simulink model "switching_controller_parallel_before_retraining"  (R2020a)
settings: Solver=FixedStepAuto  StartTime=0.0  StopTime=simulation.time_window  FixedStep=simulation.time_step  MaxStep=.2  RelTol=1e-3
model workspace (MAT data in the model file):
  PID_TRESH = 0.3
undefined symbols (not defined in the file): DiscIntNeverNeededParam
libraries: neural x36, simulink x1
(part 2 of 2)

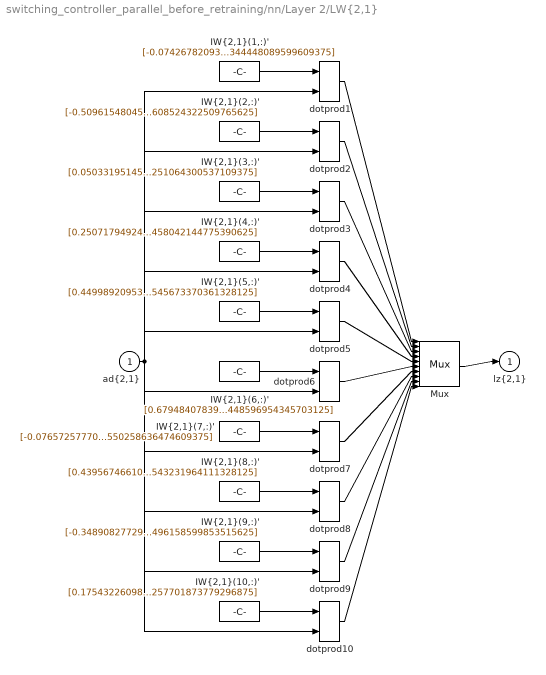
== system switching_controller_parallel_before_retraining/nn/Layer 2/LW{2,1} ==
  "ad{2,1}" : Inport  PortDimensions=20
      mask Display: e = 0.06;c1 = [120 230 180]/255;c2 = ([120 230 180]+0)/(256+128);c3 = ([120 230 180]+128)/(256+128);patch([0 1 1 0],[0 0 1 1],c1);patch([0 1 1 1-e 1-e 0+e],[0 0 1 1-e 0+e 0+e],c2);patch([0 0 1 1-e 0+e 0+e],[0 1 1 1-e 1-e 0+e],c3);plot([0 1 1 0 0],[0 0 1 1 0]);
  "IW{2,1}(1,:)'" : Constant  Value=[-0.0742678209385321530522361399562214501202106475830078125;-0.25241332220814294284849665928049944341182708740234375;0.1582652995009124208269923883563023991882801055908203125;0.0409941814809637872230041466536931693553924560546875;0.1777509687795489623507450005490682087838649749755859375;-0.56378494502083043027340636399458162486553192138671875;-0.52966898056344147160956481457105837762355804443359375;-0.5491849542615752088892122628749348223209381103515625;-0.366642992817404422822846754570491611957550048828125;-0.30113881397149777630062317257397808134555816650390625;0.36352811076936453194008436184958554804325103759765625;-0.5626667254561283915137437361408956348896026611328125;0.27233462192782542654612143451231531798839569091796875;-0.137529463271337970553531704354099929332733154296875;0.2251042526934673160265987235106877051293849945068359375;-0.267991412908181458885081838161568157374858856201171875;0.0487266727373815433654868911617086268961429595947265625;0.52897529061972725639151349241728894412517547607421875;0.08173542337008686542443314237971208058297634124755859375;-0.72183912669657279703727681408054195344448089599609375]
      mask Display: e = 0.06;c1 = [120 150 230]/255;c2 = ([120 150 230]+0)/383;c3 = ([120 150 230]+128)/383;patch([0 1 1 0],[0 0 1 1],c1);patch([0 1 1 1-e 1-e 0+e],[0 0 1 1-e 0+e 0+e],c2);patch([0 0 1 1-e 0+e 0+e],[0 1 1 1-e 1-e 0+e],c3);plot([0 1 1 0 0],[0 0 1 1 0]);disp('weights');
  "IW{2,1}(10,:)'" : Constant  Value=[0.1754322609814331357380723375172237865626811981201171875;0.33947484743859224209927560877986252307891845703125;0.322169525908290677040923810636741109192371368408203125;-0.5029839312713904053708802166511304676532745361328125;0.376908084486362648934942853884422220289707183837890625;-0.19411578487550318339316390847670845687389373779296875;-0.472436961613329098330638089464628137648105621337890625;-0.4250614998526458521155291236937046051025390625;-0.321656192995510459287089588542585261166095733642578125;0.409800051137812537671578638764913193881511688232421875;0.1634407939921007635319938344764523208141326904296875;-0.1060868965133207331152931374163017608225345611572265625;-0.417317840820639773813383044398506172001361846923828125;0.53238420036386358002999941163579933345317840576171875;-0.271228839256366149879085014617885462939739227294921875;-0.390405815950181367401938814509776420891284942626953125;-0.35866328688225135312706015611183829605579376220703125;0.394312295760493702889704081826494075357913970947265625;0.464923085316455597659768272933433763682842254638671875;0.181321777068363221285807185267913155257701873779296875]
      mask Display: e = 0.06;c1 = [120 150 230]/255;c2 = ([120 150 230]+0)/383;c3 = ([120 150 230]+128)/383;patch([0 1 1 0],[0 0 1 1],c1);patch([0 1 1 1-e 1-e 0+e],[0 0 1 1-e 0+e 0+e],c2);patch([0 0 1 1-e 0+e 0+e],[0 1 1 1-e 1-e 0+e],c3);plot([0 1 1 0 0],[0 0 1 1 0]);disp('weights');
  "IW{2,1}(2,:)'" : Constant  Value=[-0.50961548045789861749454985329066403210163116455078125;-0.253176760952781965130498065263964235782623291015625;-0.436374658893074085508345660855411551892757415771484375;-0.058776816615726999726287971270721754990518093109130859375;-0.1343536738257948837116373397293500602245330810546875;-0.53904710028970426183292374844313599169254302978515625;0.52574685179374025523202362819574773311614990234375;-0.14503214797993979612300563530880026519298553466796875;-0.41610507400117657805793669467675499618053436279296875;0.2258338290688970129149737431362154893577098846435546875;0.452630270340266649409244337221025489270687103271484375;-0.3838510809241111321199468875420279800891876220703125;-0.080043804629484960333485332739655859768390655517578125;0.086988039921783444352598735349602065980434417724609375;-0.30566584836628951649117880151607096195220947265625;0.078603298531889131961492012123926542699337005615234375;-0.2146956389255603447896447733000968582928180694580078125;-0.49159733673330541225965362173155881464481353759765625;-0.07920516278329912951416957866968004964292049407958984375;-0.2297869666393469734178012231495813466608524322509765625]
      mask Display: e = 0.06;c1 = [120 150 230]/255;c2 = ([120 150 230]+0)/383;c3 = ([120 150 230]+128)/383;patch([0 1 1 0],[0 0 1 1],c1);patch([0 1 1 1-e 1-e 0+e],[0 0 1 1-e 0+e 0+e],c2);patch([0 0 1 1-e 0+e 0+e],[0 1 1 1-e 1-e 0+e],c3);plot([0 1 1 0 0],[0 0 1 1 0]);disp('weights');
  "IW{2,1}(3,:)'" : Constant  Value=[0.050331951453894137327171875995190930552780628204345703125;-0.1980455271011341000786387667176313698291778564453125;0.5464228112888898092336376066668890416622161865234375;0.143258734343598204130643125608912669122219085693359375;0.6545378931000180866561777293100021779537200927734375;0.0029693683728794183218635538423768593929708003997802734375;0.331210089212467140296070056137978099286556243896484375;-0.05628620519114226061763162078932509757578372955322265625;0.51382712775967875895588576895534060895442962646484375;-0.21961621362080319119769455937785096466541290283203125;0.6861028831776201375447499231086112558841705322265625;0.193895474485615337822963510916451923549175262451171875;-0.25453832761822337005241934093646705150604248046875;0.45117937720722867123157584501313976943492889404296875;-0.28569063753284329454373846601811237633228302001953125;-0.50475380514631817963078219690942205488681793212890625;-0.378178164082300261039648603400564752519130706787109375;-0.03749349210638715235166529282651026733219623565673828125;0.0239248285341571442774721845125895924866199493408203125;-0.4295334690027734492190347737050615251064300537109375]
      mask Display: e = 0.06;c1 = [120 150 230]/255;c2 = ([120 150 230]+0)/383;c3 = ([120 150 230]+128)/383;patch([0 1 1 0],[0 0 1 1],c1);patch([0 1 1 1-e 1-e 0+e],[0 0 1 1-e 0+e 0+e],c2);patch([0 0 1 1-e 0+e 0+e],[0 1 1 1-e 1-e 0+e],c3);plot([0 1 1 0 0],[0 0 1 1 0]);disp('weights');
  "IW{2,1}(4,:)'" : Constant  Value=[0.25071794924415391481176129673258401453495025634765625;-0.25655473735131739676518236592528410255908966064453125;-0.125932536431736907811540504553704522550106048583984375;0.2358601050679441646362732853958732448518276214599609375;-0.50129483332140190032788495955173857510089874267578125;-0.07287292485839162725635986816996592096984386444091796875;-0.349288031403435395016998654682538472115993499755859375;0.10293619314487244265077237059813342057168483734130859375;-0.10469867031949632585341447565951966680586338043212890625;-0.398005841630075518633447018146398477256298065185546875;1.2743088847126571305778952591936103999614715576171875;0.426094930489777201643164517008699476718902587890625;0.3634133834892663283966385279200039803981781005859375;-0.0288941994596689059882077543761624838225543498992919921875;-0.30862723401891811736419413136900402605533599853515625;0.4189583770900477954768348354264162480831146240234375;-0.1382079784576591141576074051044997759163379669189453125;-0.288297871213736012219186477523180656135082244873046875;0.224223812097748720351120255145360715687274932861328125;0.06845932428237412603611034001005464233458042144775390625]
      mask Display: e = 0.06;c1 = [120 150 230]/255;c2 = ([120 150 230]+0)/383;c3 = ([120 150 230]+128)/383;patch([0 1 1 0],[0 0 1 1],c1);patch([0 1 1 1-e 1-e 0+e],[0 0 1 1-e 0+e 0+e],c2);patch([0 0 1 1-e 0+e 0+e],[0 1 1 1-e 1-e 0+e],c3);plot([0 1 1 0 0],[0 0 1 1 0]);disp('weights');
  "IW{2,1}(5,:)'" : Constant  Value=[0.449989209535755441127236053944216109812259674072265625;0.1668938640746752966048660482556442730128765106201171875;-0.1528747166922375944064782515852130018174648284912109375;-0.466413182483166377512162625862401910126209259033203125;0.319019707786719119990692661303910426795482635498046875;-0.269682605526375407389849669925752095878124237060546875;-0.286146420418946723085440453360206447541713714599609375;-0.1124570366042244862203602906447486020624637603759765625;-0.60761075348500115378413966027437709271907806396484375;-0.09832625527147524635562803041466395370662212371826171875;0.416238919016751030000023092725314199924468994140625;0.41417684214283412291734975951840169727802276611328125;0.1285238721039599629758498622322804294526576995849609375;0.04150845561035156061624462608961039222776889801025390625;-0.5181335247944744981651865600724704563617706298828125;0.024835012212249894802962302264859317801892757415771484375;-0.370454183035626993802935658095520921051502227783203125;0.260088553967631863628184873959980905055999755859375;0.437350919400649795765190219754003919661045074462890625;-0.46632501805306703079878616335918195545673370361328125]
      mask Display: e = 0.06;c1 = [120 150 230]/255;c2 = ([120 150 230]+0)/383;c3 = ([120 150 230]+128)/383;patch([0 1 1 0],[0 0 1 1],c1);patch([0 1 1 1-e 1-e 0+e],[0 0 1 1-e 0+e 0+e],c2);patch([0 0 1 1-e 0+e 0+e],[0 1 1 1-e 1-e 0+e],c3);plot([0 1 1 0 0],[0 0 1 1 0]);disp('weights');
  "IW{2,1}(6,:)'" : Constant  Value=[0.679484078395458102050952220452018082141876220703125;0.04141787402921648375553331788978539407253265380859375;-0.07852831144106568739271523327261093072593212127685546875;-0.06946291361144722731335576781930285505950450897216796875;0.5862015780018110522320284871966578066349029541015625;0.008164688663760931441881751879918738268315792083740234375;0.01267656278289677578008376457319172914139926433563232421875;0.35129857330214397936885006856755353510379791259765625;-0.281716957188827610281123270397074520587921142578125;-0.377956077447295590854281499559874646365642547607421875;0.399883631711499820671207316991058178246021270751953125;0.421701849253063698608201548267970792949199676513671875;0.38087921164733506973476551138446666300296783447265625;-0.1444822361794708687199317864724434912204742431640625;-0.3082207979968611955001733804238028824329376220703125;0.52705156187305790549402217948227189481258392333984375;0.211120738453866751971332860193797387182712554931640625;0.64083647291273748702877810501377098262310028076171875;-0.33683964993104031915294171994901262223720550537109375;0.258659389379542137277212532353587448596954345703125]
      mask Display: e = 0.06;c1 = [120 150 230]/255;c2 = ([120 150 230]+0)/383;c3 = ([120 150 230]+128)/383;patch([0 1 1 0],[0 0 1 1],c1);patch([0 1 1 1-e 1-e 0+e],[0 0 1 1-e 0+e 0+e],c2);patch([0 0 1 1-e 0+e 0+e],[0 1 1 1-e 1-e 0+e],c3);plot([0 1 1 0 0],[0 0 1 1 0]);disp('weights');
  "IW{2,1}(7,:)'" : Constant  Value=[-0.0765725777039530097756170334832859225571155548095703125;0.045295261798219167703738463615081855095922946929931640625;0.120469739157076538571544688238645903766155242919921875;0.3880656334730634426932738278992474079132080078125;-0.175604394629628013380084894379251636564731597900390625;0.1717388843781173235480963512600283138453960418701171875;0.381286326232597894136944205456529743969440460205078125;0.511569138199252648746551130898296833038330078125;0.11038162503234556777176322839295607991516590118408203125;0.6655250283685323342552919712034054100513458251953125;-0.3652469434145084736798025915049947798252105712890625;0.07177631492141227365078037792045506648719310760498046875;0.069664886066460873781380769287352450191974639892578125;-0.432032970640127411687814174001687206327915191650390625;-0.583466461683132653348593521513976156711578369140625;0.55591735512564655063982854699133895337581634521484375;-0.270067076847661013960788523036171682178974151611328125;0.382977519217001127760369172392529435455799102783203125;0.264177680981460272224836671739467419683933258056640625;-0.1612088776390406541505484483423060737550258636474609375]
      mask Display: e = 0.06;c1 = [120 150 230]/255;c2 = ([120 150 230]+0)/383;c3 = ([120 150 230]+128)/383;patch([0 1 1 0],[0 0 1 1],c1);patch([0 1 1 1-e 1-e 0+e],[0 0 1 1-e 0+e 0+e],c2);patch([0 0 1 1-e 0+e 0+e],[0 1 1 1-e 1-e 0+e],c3);plot([0 1 1 0 0],[0 0 1 1 0]);disp('weights');
  "IW{2,1}(8,:)'" : Constant  Value=[0.439567466102353698875759846487198956310749053955078125;-0.55137685168932482060455413375166244804859161376953125;-0.29550672253545806622554437126382254064083099365234375;-0.036798516056060610879274719309250940568745136260986328125;-0.2344144146160440644877098748111166059970855712890625;-0.0033479905308381983919385760373188531957566738128662109375;0.457258477431225662801494991072104312479496002197265625;0.1756065159579283940782801209934405051171779632568359375;-0.39986310942029390513852149524609558284282684326171875;0.387889234221364176402602197413216345012187957763671875;0.323256941358727456492516694197547622025012969970703125;-0.3450151758691768488773732315166853368282318115234375;0.250121520022025978224888831391581334173679351806640625;-0.331325186764646117953958537327707745134830474853515625;-0.12454398304874965408561848789759096689522266387939453125;0.33192464683260436419942607244593091309070587158203125;-0.11336549584819836933302639181420090608298778533935546875;0.4194666692769544180663388033281080424785614013671875;-0.0859583866602976198745267311096540652215480804443359375;-0.3360408023214376260767721760203130543231964111328125]
      mask Display: e = 0.06;c1 = [120 150 230]/255;c2 = ([120 150 230]+0)/383;c3 = ([120 150 230]+128)/383;patch([0 1 1 0],[0 0 1 1],c1);patch([0 1 1 1-e 1-e 0+e],[0 0 1 1-e 0+e 0+e],c2);patch([0 0 1 1-e 0+e 0+e],[0 1 1 1-e 1-e 0+e],c3);plot([0 1 1 0 0],[0 0 1 1 0]);disp('weights');
  "IW{2,1}(9,:)'" : Constant  Value=[-0.348908277292868718166829467008938081562519073486328125;-0.646467201462592289118447297369129955768585205078125;-0.422726956838112066794366228350554592907428741455078125;-0.269421098258072422293452063968288712203502655029296875;0.09081208334368238987988064536693855188786983489990234375;0.11206987819075374390731525409137248061597347259521484375;-0.438503899847936196021436217051814310252666473388671875;0.0721669692656892458604289686263655312359333038330078125;0.213677452509952570114393211042624898254871368408203125;-0.57502231817834614790996283772983588278293609619140625;-0.1320225168627740808258153037968440912663936614990234375;-0.115198136422949459767295365963946096599102020263671875;0.08326651543012160427981172006184351630508899688720703125;-0.334785851590916616604687305880361236631870269775390625;0.39577293454353934532008452151785604655742645263671875;0.46203828149677039771603404005873017013072967529296875;0.200374932292563479041547225278918631374835968017578125;0.0738423790724957729292299291046219877898693084716796875;0.61243768330698877822015901983832009136676788330078125;-0.28373973484362535746328148889006115496158599853515625]
      mask Display: e = 0.06;c1 = [120 150 230]/255;c2 = ([120 150 230]+0)/383;c3 = ([120 150 230]+128)/383;patch([0 1 1 0],[0 0 1 1],c1);patch([0 1 1 1-e 1-e 0+e],[0 0 1 1-e 0+e 0+e],c2);patch([0 0 1 1-e 0+e 0+e],[0 1 1 1-e 1-e 0+e],c3);plot([0 1 1 0 0],[0 0 1 1 0]);disp('weights');
  Mux : Mux  Inputs=10
      mask Display: e = 0.06;c1 = [120 150 230]/255;c2 = ([120 150 230]+0)/383;c3 = ([120 150 230]+128)/383;patch([0 1 1 0],[0 0 1 1],c1);patch([0 1 1 1-e 1-e 0+e],[0 0 1 1-e 0+e 0+e],c2);patch([0 0 1 1-e 0+e 0+e],[0 1 1 1-e 1-e 0+e],c3);plot([0 1 1 0 0],[0 0 1 1 0]);disp('Mux');
  dotprod{1..10} (10 alike) : neural/Weight Functions/dotprod
  "lz{2,1}" : Outport
      mask Display: e = 0.06;c1 = [120 230 180]/255;c2 = ([120 230 180]+0)/(256+128);c3 = ([120 230 180]+128)/(256+128);patch([0 1 1 0],[0 0 1 1],c1);patch([0 1 1 1-e 1-e 0+e],[0 0 1 1-e 0+e 0+e],c2);patch([0 0 1 1-e 0+e 0+e],[0 1 1 1-e 1-e 0+e],c3);plot([0 1 1 0 0],[0 0 1 1 0]);
  wires:
  "IW{2,1}(1,:)'"/1 -> dotprod1/1
  "ad{2,1}"/1 -> dotprod1/2, dotprod2/2, dotprod3/2, dotprod4/2, dotprod5/2, dotprod6/2, dotprod7/2, dotprod8/2, dotprod9/2, dotprod10/2
  dotprod1/1 -> Mux/1
  "IW{2,1}(2,:)'"/1 -> dotprod2/1
  dotprod2/1 -> Mux/2
  "IW{2,1}(3,:)'"/1 -> dotprod3/1
  dotprod3/1 -> Mux/3
  "IW{2,1}(4,:)'"/1 -> dotprod4/1
  dotprod4/1 -> Mux/4
  "IW{2,1}(5,:)'"/1 -> dotprod5/1
  dotprod5/1 -> Mux/5
  "IW{2,1}(6,:)'"/1 -> dotprod6/1
  dotprod6/1 -> Mux/6
  "IW{2,1}(7,:)'"/1 -> dotprod7/1
  dotprod7/1 -> Mux/7
  "IW{2,1}(8,:)'"/1 -> dotprod8/1
  dotprod8/1 -> Mux/8
  "IW{2,1}(9,:)'"/1 -> dotprod9/1
  dotprod9/1 -> Mux/9
  "IW{2,1}(10,:)'"/1 -> dotprod10/1
  dotprod10/1 -> Mux/10
  Mux/1 -> "lz{2,1}"/1

== system switching_controller_parallel_before_retraining/nn/Layer 3/Delays 1 ==
  "p{3}" : Inport  PortDimensions=10
      mask Display: e = 0.06;c1 = [120 230 180]/255;c2 = ([120 230 180]+0)/(256+128);c3 = ([120 230 180]+128)/(256+128);patch([0 1 1 0],[0 0 1 1],c1);patch([0 1 1 1-e 1-e 0+e],[0 0 1 1-e 0+e 0+e],c2);patch([0 0 1 1-e 0+e 0+e],[0 1 1 1-e 1-e 0+e],c3);plot([0 1 1 0 0],[0 0 1 1 0]);
  mux : Mux  Inputs=1
      mask Display: e = 0.06;c1 = [120 150 230]/255;c2 = ([120 150 230]+0)/383;c3 = ([120 150 230]+128)/383;patch([0 1 1 0],[0 0 1 1],c1);patch([0 1 1 1-e 1-e 0+e],[0 0 1 1-e 0+e 0+e],c2);patch([0 0 1 1-e 0+e 0+e],[0 1 1 1-e 1-e 0+e],c3);plot([0 1 1 0 0],[0 0 1 1 0]);disp('Mux')
  "pd{3,2}" : Outport
      mask Display: e = 0.06;c1 = [120 230 180]/255;c2 = ([120 230 180]+0)/(256+128);c3 = ([120 230 180]+128)/(256+128);patch([0 1 1 0],[0 0 1 1],c1);patch([0 1 1 1-e 1-e 0+e],[0 0 1 1-e 0+e 0+e],c2);patch([0 0 1 1-e 0+e 0+e],[0 1 1 1-e 1-e 0+e],c3);plot([0 1 1 0 0],[0 0 1 1 0]);
  wires:
  "p{3}"/1 -> mux/1
  mux/1 -> "pd{3,2}"/1

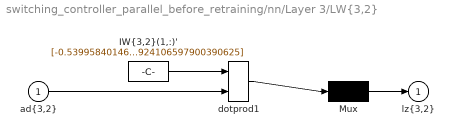
== system switching_controller_parallel_before_retraining/nn/Layer 3/LW{3,2} ==
  "ad{3,2}" : Inport  PortDimensions=10
      mask Display: e = 0.06;c1 = [120 230 180]/255;c2 = ([120 230 180]+0)/(256+128);c3 = ([120 230 180]+128)/(256+128);patch([0 1 1 0],[0 0 1 1],c1);patch([0 1 1 1-e 1-e 0+e],[0 0 1 1-e 0+e 0+e],c2);patch([0 0 1 1-e 0+e 0+e],[0 1 1 1-e 1-e 0+e],c3);plot([0 1 1 0 0],[0 0 1 1 0]);
  "IW{3,2}(1,:)'" : Constant  Value=[-0.53995840146214668653357193761621601879596710205078125;0.447069122341665903253016267626662738621234893798828125;0.5766855779899859868464773171581327915191650390625;0.83408591078783589356504535317071713507175445556640625;0.0792445839882247593521924500237219035625457763671875;-0.32847391934336656049708835780620574951171875;-0.713046634792105837874487406224943697452545166015625;0.6129975272120213869442295617773197591304779052734375;-0.150298728108551438165108038447215221822261810302734375;0.307691133356994550585028491695993579924106597900390625]
      mask Display: e = 0.06;c1 = [120 150 230]/255;c2 = ([120 150 230]+0)/383;c3 = ([120 150 230]+128)/383;patch([0 1 1 0],[0 0 1 1],c1);patch([0 1 1 1-e 1-e 0+e],[0 0 1 1-e 0+e 0+e],c2);patch([0 0 1 1-e 0+e 0+e],[0 1 1 1-e 1-e 0+e],c3);plot([0 1 1 0 0],[0 0 1 1 0]);disp('weights');
  Mux : Mux  Inputs=1
      mask Display: e = 0.06;c1 = [120 150 230]/255;c2 = ([120 150 230]+0)/383;c3 = ([120 150 230]+128)/383;patch([0 1 1 0],[0 0 1 1],c1);patch([0 1 1 1-e 1-e 0+e],[0 0 1 1-e 0+e 0+e],c2);patch([0 0 1 1-e 0+e 0+e],[0 1 1 1-e 1-e 0+e],c3);plot([0 1 1 0 0],[0 0 1 1 0]);disp('Mux');
  dotprod1 : neural/Weight Functions/dotprod
  "lz{3,2}" : Outport
      mask Display: e = 0.06;c1 = [120 230 180]/255;c2 = ([120 230 180]+0)/(256+128);c3 = ([120 230 180]+128)/(256+128);patch([0 1 1 0],[0 0 1 1],c1);patch([0 1 1 1-e 1-e 0+e],[0 0 1 1-e 0+e 0+e],c2);patch([0 0 1 1-e 0+e 0+e],[0 1 1 1-e 1-e 0+e],c3);plot([0 1 1 0 0],[0 0 1 1 0]);
  wires:
  "IW{3,2}(1,:)'"/1 -> dotprod1/1
  "ad{3,2}"/1 -> dotprod1/2
  dotprod1/1 -> Mux/1
  Mux/1 -> "lz{3,2}"/1

== stateflow chart switching_controller_parallel_before_retraining/SwitchingController ==
  state STEADY
    entry: u = 0;
  state P
    du:
    u = p_control(e);
    state u = p_control(e) [function]
  state PID
    du:
    u = pid_control(e);
    state u = pid_control(e) [function]
  (default) -> STEADY
  STEADY -> P : [e > 0.01]
  P -> PID : [e < PID_TRESH]
  data: e function_input; u function_output; e function_input; u function_output; e input; u output double; PID output boolean; PID_TRESH parameter; P output boolean
